simulink model "transystem2"  (Simulink 10.0)
settings: Solver=ode15s  StartTime=0.0  StopTime=1  RelTol=1e-3  AbsTol=1e-6
libraries: powerlib x86, powerlib_extras x4
settings Model: Creator=Dr. Lotfifard  LastModifiedBy=bae_rashid  ExtModeTrigMode=oneshot  ExtModeArmWhenConnect=off
settings SolverCC: AutoScaleAbsTol=off
settings DataIOCC: SignalLoggingSaveFormat=ModelDataLogs
settings OptimizationCC: BlockReduction=off  BooleanDataType=off  ExpressionDepthLimit=2147483647
settings DebuggingCC: SaveWithParameterizedLinksMsg=none  SignalResolutionControl=TryResolveAllWithWarning  MultiTaskDSMMsg=warning  MultiTaskCondExecSysMsg=none  FcnCallInpInsideContextMsg=warning  StateNameClashWarn=warning
settings HardwareCC: TargetUnknown=on
settings GRTTargetCC: GeneratePreprocessorConditionals=Disable all
settings ConfigComp: CovExternalEMLEnable=off
settings SimscapeCC: SimscapeNormalizeSystem=off

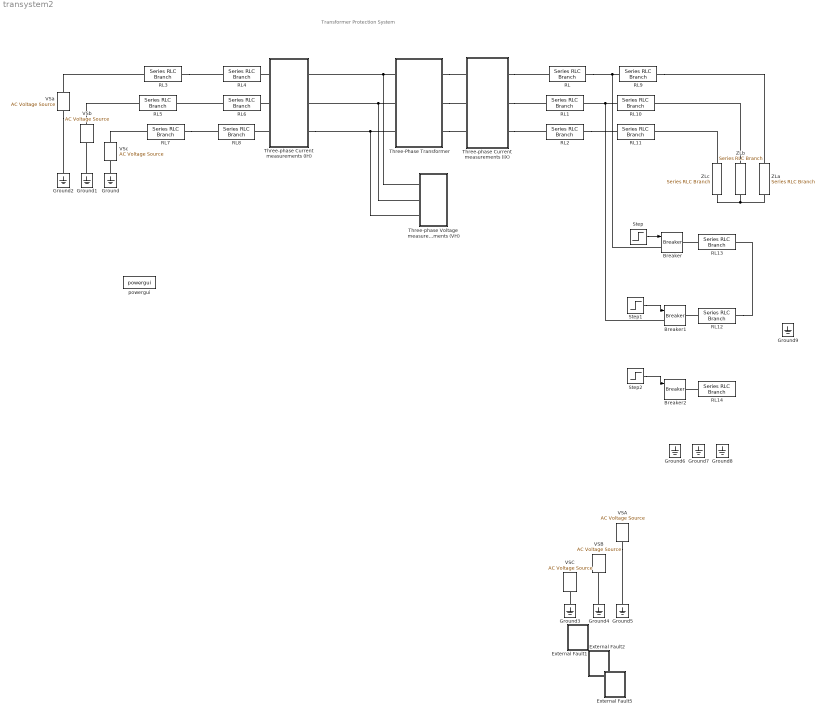
== system transystem2 ==
  note: Transformer Protection System
  Breaker : powerlib/Elements/Breaker  Tag=PoWeRsYsTeMbLoCk  InitialState=0  SwitchingTimes="[ 1/60  5/60 ]"  External=on  BreakerResistance=0.01  SnubberResistance=1e6  SnubberCapacitance=inf  Measurements=None  MoreParameters=off  NoBreakLoop=off
      settings: SourceProductName=Simscape Electrical
  Breaker1 : powerlib/Elements/Breaker  Tag=PoWeRsYsTeMbLoCk  InitialState=0  SwitchingTimes="[ 1/60  5/60 ]"  External=on  BreakerResistance=0.01  SnubberResistance=1e6  SnubberCapacitance=inf  Measurements=None  MoreParameters=off  NoBreakLoop=off
      settings: SourceProductName=Simscape Electrical
  Breaker2 : powerlib/Elements/Breaker  Tag=PoWeRsYsTeMbLoCk  InitialState=0  SwitchingTimes="[ 1/60  5/60 ]"  External=on  BreakerResistance=0.01  SnubberResistance=1e6  SnubberCapacitance=inf  Measurements=None  MoreParameters=off  NoBreakLoop=off
      settings: SourceProductName=Simscape Electrical
  External Fault1 : Subsystem  mask(Fault){RF=1, tf=0.5}
      mask prompts: RF "Resistance [ohm]"; tf "Time [sec]"
      mask Display: plot(0,0,100,100,[44,47,56,38,50],[23,8,64,44,97],[56,47],[25,8])
  External Fault2 : Subsystem  mask(Fault){RF=1, tf=0.5}
      mask prompts: RF "Resistance [ohm]"; tf "Time [sec]"
      mask Display: plot(0,0,100,100,[44,47,56,38,50],[23,8,64,44,97],[56,47],[25,8])
  External Fault5 : Subsystem  mask(Fault){RF=1, tf=0.5}
      mask prompts: RF "Resistance [ohm]"; tf "Time [sec]"
      mask Display: plot(0,0,100,100,[44,47,56,38,50],[23,8,64,44,97],[56,47],[25,8])
  Ground{,1..9} (10 alike) : powerlib/Elements/Ground  LConnTagsString=a
      settings: SourceProductName=Simscape Electrical
  RL{,1..2,9..11} (6 alike) : powerlib/Elements/Series RLC Branch  LConnTagsString=__new0  RConnTagsString=__new0  BranchType=RL  Resistance=10  Inductance=0.033  SetiL0=off  InitialCurrent=0  Capacitance=1e-6  Setx0=off  InitialVoltage=0  Measurements=None
      settings: SourceProductName=Simscape Electrical
  RL12 : powerlib/Elements/Series RLC Branch  LConnTagsString=__new0  RConnTagsString=__new0  BranchType=RL  Resistance=1  Inductance=0.000001/(2*pi*60)/(2*pi*60)  SetiL0=off  InitialCurrent=0  Capacitance=1e-6  Setx0=off  InitialVoltage=0  Measurements=None
      settings: SourceProductName=Simscape Electrical
  RL13 : powerlib/Elements/Series RLC Branch  LConnTagsString=__new0  RConnTagsString=__new0  BranchType=RL  Resistance=1  Inductance=0.000001/(2*pi*60)  SetiL0=off  InitialCurrent=0  Capacitance=1e-6  Setx0=off  InitialVoltage=0  Measurements=None
      settings: SourceProductName=Simscape Electrical
  RL14 : powerlib/Elements/Series RLC Branch  LConnTagsString=__new0  RConnTagsString=__new0  BranchType=RL  Resistance=1  Inductance=0.000001/(2*pi*60)/(2*pi*60)  SetiL0=off  InitialCurrent=0  Capacitance=1e-6  Setx0=off  InitialVoltage=0  Measurements=None
      settings: SourceProductName=Simscape Electrical
  RL{3..8} (6 alike) : powerlib/Elements/Series RLC Branch  LConnTagsString=__new0  RConnTagsString=__new0  BranchType=RL  Resistance=6  Inductance=0.09  SetiL0=off  InitialCurrent=0  Capacitance=1e-6  Setx0=off  InitialVoltage=0  Measurements=None
      settings: SourceProductName=Simscape Electrical
  Step : Step  Time=0.5
  Step1 : Step  Time=0.5
  Step2 : Step  Time=0.5
  Three-Phase Transformer : Subsystem
  Three-phase Current  measurements (IH) : Subsystem
  Three-phase Current  measurements (IX) : Subsystem
  Three-phase Voltage  measurements (VH) : Subsystem
  VSA : powerlib/Electrical Sources/AC Voltage Source  Amplitude=3.8e3/sqrt(3)*sqrt(2)  Phase=0  Frequency=60  SampleTime=0  Measurements=None  BusType=swing  Pref=10e3  Qref=0  Qmin=-inf  Qmax=+inf
      settings: SourceProductName=Simscape Electrical
  VSB : powerlib/Electrical Sources/AC Voltage Source  Amplitude=3.8e3/sqrt(3)*sqrt(2)  Phase=-120  Frequency=60  SampleTime=0  Measurements=None  BusType=swing  Pref=10e3  Qref=0  Qmin=-inf  Qmax=+inf
      settings: SourceProductName=Simscape Electrical
  VSC : powerlib/Electrical Sources/AC Voltage Source  Amplitude=3.8e3/sqrt(3)*sqrt(2)  Phase=120  Frequency=60  SampleTime=0  Measurements=None  BusType=swing  Pref=10e3  Qref=0  Qmin=-inf  Qmax=+inf
      settings: SourceProductName=Simscape Electrical
  VSa : powerlib/Electrical Sources/AC Voltage Source  Amplitude=315e3/sqrt(3)*sqrt(2)  Phase=0  Frequency=60  SampleTime=0  Measurements=None  BusType=swing  Pref=10e3  Qref=0  Qmin=-inf  Qmax=+inf
      settings: SourceProductName=Simscape Electrical
  VSb : powerlib/Electrical Sources/AC Voltage Source  Amplitude=315e3/sqrt(3)*sqrt(2)  Phase=-120  Frequency=60  SampleTime=0  Measurements=None  BusType=swing  Pref=10e3  Qref=0  Qmin=-inf  Qmax=+inf
      settings: SourceProductName=Simscape Electrical
  VSc : powerlib/Electrical Sources/AC Voltage Source  Amplitude=315e3/sqrt(3)*sqrt(2)  Phase=120  Frequency=60  SampleTime=0  Measurements=None  BusType=swing  Pref=10e3  Qref=0  Qmin=-inf  Qmax=+inf
      settings: SourceProductName=Simscape Electrical
  ZLa : powerlib/Elements/Series RLC Branch  LConnTagsString=__new0  RConnTagsString=__new0  BranchType=RL  Resistance=300  Inductance=450/(2*pi*60)  SetiL0=off  InitialCurrent=0  Capacitance=1.0  Setx0=off  InitialVoltage=0  Measurements=None
      settings: SourceProductName=Simscape Electrical
  ZLb : powerlib/Elements/Series RLC Branch  LConnTagsString=__new0  RConnTagsString=__new0  BranchType=RL  Resistance=300  Inductance=450/(2*pi*60)  SetiL0=off  InitialCurrent=0  Capacitance=1.0  Setx0=off  InitialVoltage=0  Measurements=None
      settings: SourceProductName=Simscape Electrical
  ZLc : powerlib/Elements/Series RLC Branch  LConnTagsString=__new0  RConnTagsString=__new0  BranchType=RL  Resistance=300  Inductance=450/(2*pi*60)  SetiL0=off  InitialCurrent=0  Capacitance=1.0  Setx0=off  InitialVoltage=0  Measurements=None
      settings: SourceProductName=Simscape Electrical
  powergui : powerlib/powergui  SimulationMode=Continuous  SampleTime=0  frequency=60  Iterations=50  frequencyindice=60  Pbase=100e6  ErrMax=1e-4  UnitsV=kV  UnitsW=MW  buscounter=0  FunctionMessages=off  echomessages=off  EnableUseOfTLC=off  CurrentSourceSwitches=on  DisableSnubberDevices=off  DisableRonSwitches=off  DisableVfSwitches=off  DisplayEquations=off  AutomaticDiscreteSolvers=off  SolverType=Tustin/Backward Euler (TBE)  Interpol=off  ExternalGateDelay=off  methode=off  Ts=0  x0status=blocks  SPID=off  SwTol=0  HookPort=off  NonlinearTolerance=0  nMaxIteration=15  ContinueOnMaxIteration=off  RestoreLinks=warning  ResistiveCurrentMeasurement=off  Frange=[0:2:500]  Ylog=off  Xlog=on  ShowGrid=off  save=off  variable=ZData  structure=0  ZoomFFT=on  StartTime=0.0  cycles=1  DisplayStyle=1  fundamental=60  FreqAxis=off  MaxFrequency=1000  frequencyindicesteady=1  RmsSteady=1  display=off
      settings: SourceProductName=Simscape Electrical
  wires:
  Step/1 -> Breaker/1
  Step1/1 -> Breaker1/1
  Step2/1 -> Breaker2/1
  connections:
  Ground/LConn1 -- VSc/LConn1
  Ground1/LConn1 -- VSb/LConn1
  VSa/LConn1 -- Ground2/LConn1
  RL5/LConn1 -- VSb/RConn1
  Three-phase Current  measurements (IH)/LConn2 -- RL6/RConn1
  Three-phase Current  measurements (IH)/LConn3 -- RL8/RConn1
  Three-phase Current  measurements (IH)/LConn1 -- RL4/RConn1
  VSa/RConn1 -- RL3/LConn1
  RL6/LConn1 -- RL5/RConn1
  RL3/RConn1 -- RL4/LConn1
  RL7/RConn1 -- RL8/LConn1
  RL7/LConn1 -- VSc/RConn1
  RL10/LConn1 -- Breaker1/LConn1 -- RL1/RConn1
  RL/RConn1 -- Breaker/LConn1 -- RL9/LConn1
  RL2/RConn1 -- RL11/LConn1
  Ground3/LConn1 -- VSC/LConn1
  Ground4/LConn1 -- VSB/LConn1
  VSA/LConn1 -- Ground5/LConn1
  Three-Phase Transformer/LConn2 -- Three-phase Current  measurements (IH)/RConn2 -- Three-phase Voltage  measurements (VH)/LConn2
  Three-Phase Transformer/LConn1 -- Three-phase Current  measurements (IH)/RConn1 -- Three-phase Voltage  measurements (VH)/LConn1
  Three-Phase Transformer/RConn1 -- Three-phase Current  measurements (IX)/LConn1
  Three-phase Current  measurements (IH)/RConn3 -- Three-Phase Transformer/LConn3 -- Three-phase Voltage  measurements (VH)/LConn3
  Three-Phase Transformer/RConn3 -- Three-phase Current  measurements (IX)/LConn3
  Three-Phase Transformer/RConn2 -- Three-phase Current  measurements (IX)/LConn2
  ZLc/RConn1 -- ZLa/RConn1 -- ZLb/RConn1
  Three-phase Current  measurements (IX)/RConn3 -- RL2/LConn1
  Three-phase Current  measurements (IX)/RConn2 -- RL1/LConn1
  Three-phase Current  measurements (IX)/RConn1 -- RL/LConn1
  ZLb/LConn1 -- RL10/RConn1
  ZLc/LConn1 -- RL11/RConn1
  RL9/RConn1 -- ZLa/LConn1
  RL13/LConn1 -- Breaker/RConn1
  RL12/LConn1 -- Breaker1/RConn1
  RL14/LConn1 -- Breaker2/RConn1
  RL12/RConn1 -- RL13/RConn1

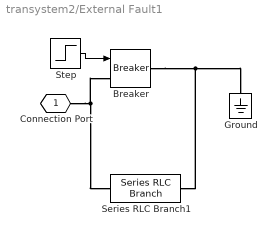
== system transystem2/External Fault1 ==
  Breaker : powerlib/Elements/Breaker  Tag=PoWeRsYsTeMbLoCk  InitialState=0  SwitchingTimes="[ 1/60  5/60 ]"  External=on  BreakerResistance=0.01  SnubberResistance=1e6  SnubberCapacitance=inf  Measurements=None  MoreParameters=off  NoBreakLoop=off
      settings: SourceProductName=Simscape Electrical
  Ground : powerlib/Elements/Ground  LConnTagsString=a
      settings: SourceProductName=Simscape Electrical
  Series RLC Branch1 : powerlib/Elements/Series RLC Branch  LConnTagsString=__new0  RConnTagsString=__new0  BranchType=RLC  Resistance=1  Inductance=1e-3  SetiL0=off  InitialCurrent=0  Capacitance=1e-6  Setx0=off  InitialVoltage=0  Measurements=None
      settings: SourceProductName=Simscape Electrical
  Step : Step  Time=tf
  Connection Port : PMIOPort  Tag=PMCPort  Side=Left
  wires:
  Step/1 -> Breaker/1
  connections:
  Breaker/RConn1 -- Ground/LConn1 -- Series RLC Branch1/RConn1
  Connection Port/RConn1 -- Breaker/LConn1 -- Series RLC Branch1/LConn1

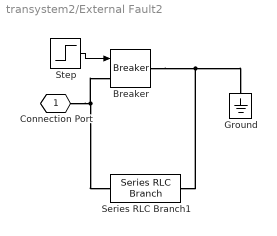
== system transystem2/External Fault2 ==
  Breaker : powerlib/Elements/Breaker  Tag=PoWeRsYsTeMbLoCk  InitialState=0  SwitchingTimes="[ 1/60  5/60 ]"  External=on  BreakerResistance=0.01  SnubberResistance=1e6  SnubberCapacitance=inf  Measurements=None  MoreParameters=off  NoBreakLoop=off
      settings: SourceProductName=Simscape Electrical
  Ground : powerlib/Elements/Ground  LConnTagsString=a
      settings: SourceProductName=Simscape Electrical
  Series RLC Branch1 : powerlib/Elements/Series RLC Branch  LConnTagsString=__new0  RConnTagsString=__new0  BranchType=RLC  Resistance=1  Inductance=1e-3  SetiL0=off  InitialCurrent=0  Capacitance=1e-6  Setx0=off  InitialVoltage=0  Measurements=None
      settings: SourceProductName=Simscape Electrical
  Step : Step  Time=tf
  Connection Port : PMIOPort  Tag=PMCPort  Side=Left
  wires:
  Step/1 -> Breaker/1
  connections:
  Breaker/RConn1 -- Ground/LConn1 -- Series RLC Branch1/RConn1
  Connection Port/RConn1 -- Breaker/LConn1 -- Series RLC Branch1/LConn1

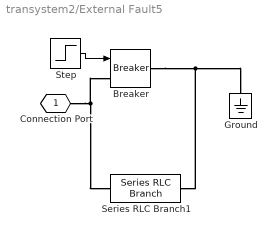
== system transystem2/External Fault5 ==
  Breaker : powerlib/Elements/Breaker  Tag=PoWeRsYsTeMbLoCk  InitialState=0  SwitchingTimes="[ 1/60  5/60 ]"  External=on  BreakerResistance=0.01  SnubberResistance=1e6  SnubberCapacitance=inf  Measurements=None  MoreParameters=off  NoBreakLoop=off
      settings: SourceProductName=Simscape Electrical
  Ground : powerlib/Elements/Ground  LConnTagsString=a
      settings: SourceProductName=Simscape Electrical
  Series RLC Branch1 : powerlib/Elements/Series RLC Branch  LConnTagsString=__new0  RConnTagsString=__new0  BranchType=RLC  Resistance=1  Inductance=1e-3  SetiL0=off  InitialCurrent=0  Capacitance=1e-6  Setx0=off  InitialVoltage=0  Measurements=None
      settings: SourceProductName=Simscape Electrical
  Step : Step  Time=tf
  Connection Port : PMIOPort  Tag=PMCPort  Side=Left
  wires:
  Step/1 -> Breaker/1
  connections:
  Breaker/RConn1 -- Ground/LConn1 -- Series RLC Branch1/RConn1
  Connection Port/RConn1 -- Breaker/LConn1 -- Series RLC Branch1/LConn1

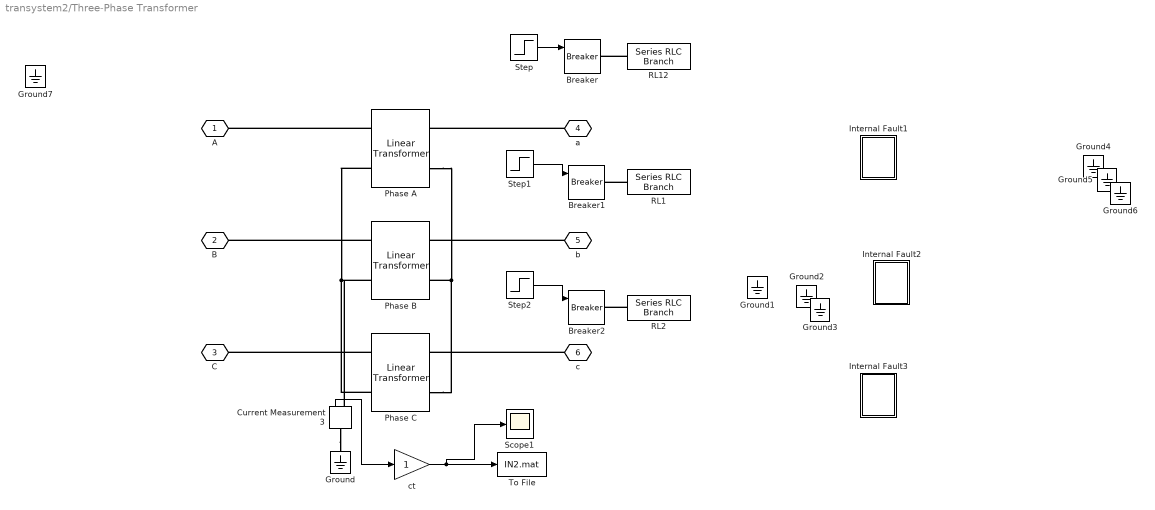
== system transystem2/Three-Phase Transformer ==
  Breaker : powerlib/Elements/Breaker  Tag=PoWeRsYsTeMbLoCk  InitialState=0  SwitchingTimes="[ 1/60  5/60 ]"  External=on  BreakerResistance=0.01  SnubberResistance=1e6  SnubberCapacitance=inf  Measurements=None  MoreParameters=off  NoBreakLoop=off
      settings: SourceProductName=Simscape Electrical
  Breaker1 : powerlib/Elements/Breaker  Tag=PoWeRsYsTeMbLoCk  InitialState=0  SwitchingTimes="[ 1/60  5/60 ]"  External=on  BreakerResistance=0.01  SnubberResistance=1e6  SnubberCapacitance=inf  Measurements=None  MoreParameters=off  NoBreakLoop=off
      settings: SourceProductName=Simscape Electrical
  Breaker2 : powerlib/Elements/Breaker  Tag=PoWeRsYsTeMbLoCk  InitialState=0  SwitchingTimes="[ 1/60  5/60 ]"  External=on  BreakerResistance=0.01  SnubberResistance=1e6  SnubberCapacitance=inf  Measurements=None  MoreParameters=off  NoBreakLoop=off
      settings: SourceProductName=Simscape Electrical
  Current Measurement3 : powerlib/Measurements/Current Measurement  PhasorSimulation=off  OutputType=Complex  PSBequivalent=0
      settings: SourceProductName=Simscape Electrical
  Ground{,1..7} (8 alike) : powerlib/Elements/Ground  LConnTagsString=a
      settings: SourceProductName=Simscape Electrical
  Internal Fault1 : Subsystem  mask(Fault){RF=1, tf=0.5}
      mask prompts: RF "Resistance [ohm]"; tf "Time [sec]"
      mask Display: plot(0,0,100,100,[44,47,56,38,50],[23,8,64,44,97],[56,47],[25,8])
  Internal Fault2 : Subsystem  mask(Fault){RF=1, tf=0.5}
      mask prompts: RF "Resistance [ohm]"; tf "Time [sec]"
      mask Display: plot(0,0,100,100,[44,47,56,38,50],[23,8,64,44,97],[56,47],[25,8])
  Internal Fault3 : Subsystem  mask(Fault){RF=1, tf=0.5}
      mask prompts: RF "Resistance [ohm]"; tf "Time [sec]"
      mask Display: plot(0,0,100,100,[44,47,56,38,50],[23,8,64,44,97],[56,47],[25,8])
  Phase A : powerlib/Elements/Linear Transformer  UNITS=pu  NominalPower=[ 300e6 60 ]  winding1="[ 315e3  0.0025  0.1 ]"  winding2="[ 13.8e3  0.0025  0.1 ]"  ThreeWindings=off  winding3=[ 315e3 0.002 0.08 ]  RmLm=[ 1e6 inf ]  Measurements=None  DataType=off
      settings: SourceProductName=Simscape Electrical
  Phase B : powerlib/Elements/Linear Transformer  UNITS=pu  NominalPower=[ 300e6 60 ]  winding1="[ 315e3  0.0025  0.1 ]"  winding2="[ 13.8e3  0.0025  0.1 ]"  ThreeWindings=off  winding3=[ 315e3 0.002 0.08 ]  RmLm=[ 1e6 inf ]  Measurements=None  DataType=off
      settings: SourceProductName=Simscape Electrical
  Phase C : powerlib/Elements/Linear Transformer  UNITS=pu  NominalPower=[ 300e6 60 ]  winding1="[ 315e3  0.0025  0.1 ]"  winding2="[ 13.8e3  0.0025  0.1 ]"  ThreeWindings=off  winding3=[ 315e3 0.002 0.08 ]  RmLm=[1e6 inf ]  Measurements=None  DataType=off
      settings: SourceProductName=Simscape Electrical
  RL1 : powerlib/Elements/Series RLC Branch  LConnTagsString=__new0  RConnTagsString=__new0  BranchType=RL  Resistance=1.5  Inductance=2/(2*pi*60)  SetiL0=off  InitialCurrent=0  Capacitance=1e-6  Setx0=off  InitialVoltage=0  Measurements=None
      settings: SourceProductName=Simscape Electrical
  RL12 : powerlib/Elements/Series RLC Branch  LConnTagsString=__new0  RConnTagsString=__new0  BranchType=RL  Resistance=1.5  Inductance=2/(2*pi*60)  SetiL0=off  InitialCurrent=0  Capacitance=1e-6  Setx0=off  InitialVoltage=0  Measurements=None
      settings: SourceProductName=Simscape Electrical
  RL2 : powerlib/Elements/Series RLC Branch  LConnTagsString=__new0  RConnTagsString=__new0  BranchType=RL  Resistance=1.5  Inductance=2/(2*pi*60)  SetiL0=off  InitialCurrent=0  Capacitance=1e-6  Setx0=off  InitialVoltage=0  Measurements=None
      settings: SourceProductName=Simscape Electrical
  Scope1 : Scope
  Step : Step  Time=0.5
  Step1 : Step  Time=0.5
  Step2 : Step  Time=0.5
  To File : ToFile  Filename=IN2.mat  MatrixName=iha
  ct : Gain  SaturateOnIntegerOverflow=on  OutDataTypeStr=Inherit: Same as input  ParamDataTypeStr=Inherit: Same as input
  A : PMIOPort  Tag=PMCPort  Side=Left
  B : PMIOPort  Tag=PMCPort  Port=2  Side=Left
  C : PMIOPort  Tag=PMCPort  Port=3  Side=Left
  a : PMIOPort  Tag=PMCPort  Port=4  Side=Right
  b : PMIOPort  Tag=PMCPort  Port=5  Side=Right
  c : PMIOPort  Tag=PMCPort  Port=6  Side=Right
  wires:
  ct/1 -> Scope1/1, To File/1
  Current Measurement3/1 -> ct/1
  Step/1 -> Breaker/1
  Step1/1 -> Breaker1/1
  Step2/1 -> Breaker2/1
  connections:
  b/RConn1 -- Phase B/RConn1
  Phase B/LConn1 -- B/RConn1
  c/RConn1 -- Phase C/RConn1
  Phase B/LConn2 -- Current Measurement3/RConn1 -- Phase C/LConn2 -- Phase A/LConn2
  a/RConn1 -- Phase A/RConn1
  Phase C/LConn1 -- C/RConn1
  Phase A/LConn1 -- A/RConn1
  Current Measurement3/LConn1 -- Ground/LConn1
  Phase A/RConn2 -- Phase C/RConn2 -- Phase B/RConn2
  RL12/LConn1 -- Breaker/RConn1
  RL1/LConn1 -- Breaker1/RConn1
  RL2/LConn1 -- Breaker2/RConn1

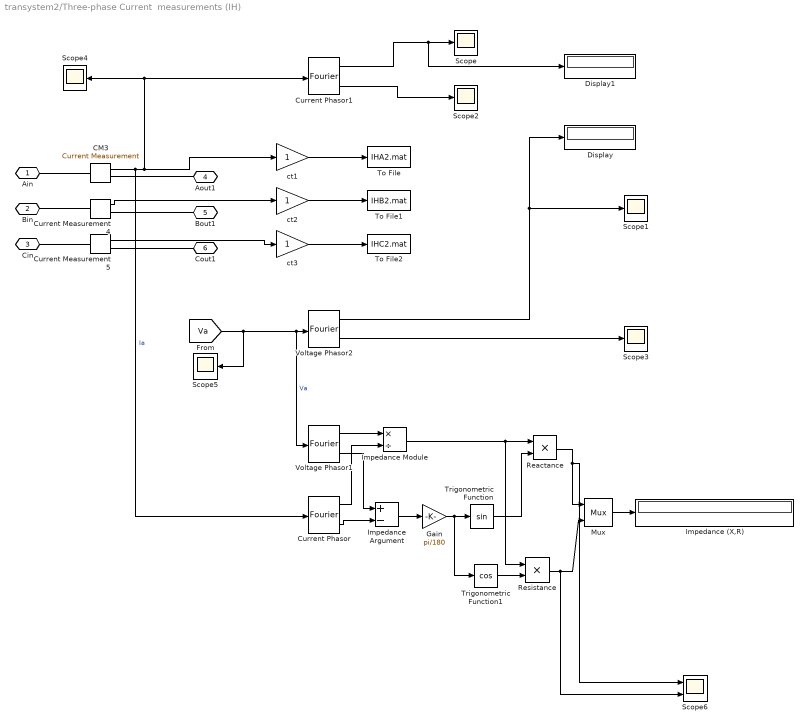
== system transystem2/Three-phase Current  measurements (IH) ==
  CM3 : powerlib/Measurements/Current Measurement  PhasorSimulation=off  OutputType=Complex  PSBequivalent=0
      settings: SourceProductName=Simscape Electrical
  Current Phasor : powerlib_extras/Measurements/Fourier  f1=60  n=1
      settings: SourceProductName=Simscape Electrical  SourceProductBaseCode=PS
  Current Phasor1 : powerlib_extras/Measurements/Fourier  f1=60  n=1
      settings: SourceProductName=Simscape Electrical  SourceProductBaseCode=PS
  Current Measurement4 : powerlib/Measurements/Current Measurement  PhasorSimulation=off  OutputType=Complex  PSBequivalent=0
      settings: SourceProductName=Simscape Electrical
  Current Measurement5 : powerlib/Measurements/Current Measurement  PhasorSimulation=off  OutputType=Complex  PSBequivalent=0
      settings: SourceProductName=Simscape Electrical
  Display : Display
      settings: Format=bank  Decimation=2
  Display1 : Display
      settings: Decimation=2
  Gain : Gain  Gain=pi/180  SaturateOnIntegerOverflow=on  OutDataTypeStr=Inherit: Same as input  ParamDataTypeStr=Inherit: Same as input
  Impedance Argument : Sum  Inputs=+-  SaturateOnIntegerOverflow=on  InputSameDT=on  OutDataTypeStr=Inherit: Same as first input
  Impedance Module : Product  Inputs=*/  SaturateOnIntegerOverflow=on  RndMeth=Zero  InputSameDT=on  OutDataTypeStr=Inherit: Same as first input
  Impedance (X,R) : Display
      settings: Format=bank
  Mux : Mux  Inputs=2
  Reactance : Product  Inputs=**  SaturateOnIntegerOverflow=on  RndMeth=Zero  InputSameDT=on  OutDataTypeStr=Inherit: Same as first input
  Resistance : Product  Inputs=**  SaturateOnIntegerOverflow=on  RndMeth=Zero  InputSameDT=on  OutDataTypeStr=Inherit: Same as first input
  Scope{,1..5} (6 alike) : Scope
  Scope6 : Scope  NumInputPorts=2
  To File : ToFile  Filename=IHA2.mat  MatrixName=iha
  To File1 : ToFile  Filename=IHB2.mat  MatrixName=ihb
  To File2 : ToFile  Filename=IHC2.mat  MatrixName=ihc
  Trigonometric Function : Trigonometry
  Trigonometric Function1 : Trigonometry  Operator=cos
  Voltage Phasor1 : powerlib_extras/Measurements/Fourier  f1=60  n=1
      settings: SourceProductName=Simscape Electrical  SourceProductBaseCode=PS
  Voltage Phasor2 : powerlib_extras/Measurements/Fourier  f1=60  n=1
      settings: SourceProductName=Simscape Electrical  SourceProductBaseCode=PS
  ct1 : Gain  SaturateOnIntegerOverflow=on  OutDataTypeStr=Inherit: Same as input  ParamDataTypeStr=Inherit: Same as input
  ct2 : Gain  SaturateOnIntegerOverflow=on  OutDataTypeStr=Inherit: Same as input  ParamDataTypeStr=Inherit: Same as input
  ct3 : Gain  SaturateOnIntegerOverflow=on  OutDataTypeStr=Inherit: Same as input  ParamDataTypeStr=Inherit: Same as input
  Ain : PMIOPort  Side=Left
  Bin : PMIOPort  Port=2  Side=Left
  Cin : PMIOPort  Port=3  Side=Left
  Aout1 : PMIOPort  Port=4  Side=Right
  Bout1 : PMIOPort  Port=5  Side=Right
  Cout1 : PMIOPort  Port=6  Side=Right
  wires:
  ct2/1 -> To File1/1
  ct3/1 -> To File2/1
  Current Measurement4/1 -> ct2/1
  Current Measurement5/1 -> ct3/1
  ct1/1 -> To File/1
  CM3/1 -> Current Phasor/1, Scope4/1, Current Phasor1/1, ct1/1  "Ia"
  Current Phasor1/1 -> Display1/1, Scope/1
  Current Phasor1/2 -> Scope2/1
  Resistance/1 -> Scope6/2, Mux/2
  Current Phasor/1 -> Impedance Module/2
  Mux/1 -> Impedance (X,R)/1
  Current Phasor/2 -> Impedance Argument/2
  Trigonometric Function1/1 -> Resistance/2
  Impedance Argument/1 -> Gain/1
  Voltage Phasor1/2 -> Impedance Argument/1
  Impedance Module/1 -> Reactance/1, Resistance/1
  Trigonometric Function/1 -> Reactance/2
  Gain/1 -> Trigonometric Function/1, Trigonometric Function1/1
  Reactance/1 -> Scope6/1, Mux/1
  Voltage Phasor1/1 -> Impedance Module/1
  [Va] -> Scope5/1, Voltage Phasor1/1, Voltage Phasor2/1  "Va"
  Voltage Phasor2/1 -> Display/1, Scope1/1
  Voltage Phasor2/2 -> Scope3/1
  connections:
  Current Measurement4/RConn1 -- Bout1/RConn1
  CM3/LConn1 -- Ain/RConn1
  Current Measurement5/LConn1 -- Cin/RConn1
  CM3/RConn1 -- Aout1/RConn1
  Current Measurement4/LConn1 -- Bin/RConn1
  Current Measurement5/RConn1 -- Cout1/RConn1

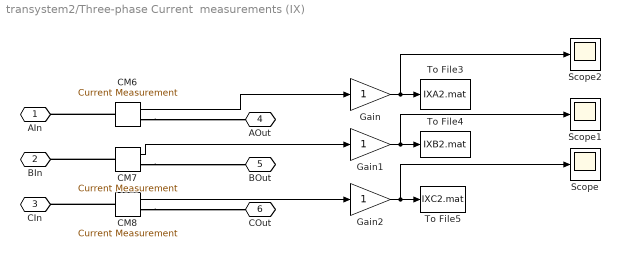
== system transystem2/Three-phase Current  measurements (IX) ==
  CM6 : powerlib/Measurements/Current Measurement  PhasorSimulation=off  OutputType=Complex  PSBequivalent=0
      settings: SourceProductName=Simscape Electrical
  CM7 : powerlib/Measurements/Current Measurement  PhasorSimulation=off  OutputType=Complex  PSBequivalent=0
      settings: SourceProductName=Simscape Electrical
  CM8 : powerlib/Measurements/Current Measurement  PhasorSimulation=off  OutputType=Complex  PSBequivalent=0
      settings: SourceProductName=Simscape Electrical
  Gain : Gain  SaturateOnIntegerOverflow=on  OutDataTypeStr=Inherit: Same as input  ParamDataTypeStr=Inherit: Same as input
  Gain1 : Gain  SaturateOnIntegerOverflow=on  OutDataTypeStr=Inherit: Same as input  ParamDataTypeStr=Inherit: Same as input
  Gain2 : Gain  SaturateOnIntegerOverflow=on  OutDataTypeStr=Inherit: Same as input  ParamDataTypeStr=Inherit: Same as input
  Scope : Scope
  Scope1 : Scope
  Scope2 : Scope
  To File3 : ToFile  Filename=IXA2.mat  MatrixName=ixa
  To File4 : ToFile  Filename=IXB2.mat  MatrixName=ixb
  To File5 : ToFile  Filename=IXC2.mat  MatrixName=ixc
  AIn : PMIOPort  Side=Left
  BIn : PMIOPort  Port=2  Side=Left
  CIn : PMIOPort  Port=3  Side=Left
  AOut : PMIOPort  Port=4  Side=Right
  BOut : PMIOPort  Port=5  Side=Right
  COut : PMIOPort  Port=6  Side=Right
  wires:
  Gain2/1 -> To File5/1, Scope/1
  Gain1/1 -> To File4/1, Scope1/1
  Gain/1 -> To File3/1, Scope2/1
  CM7/1 -> Gain1/1
  CM6/1 -> Gain/1
  CM8/1 -> Gain2/1
  connections:
  CM7/RConn1 -- BOut/RConn1
  CM6/LConn1 -- AIn/RConn1
  CM6/RConn1 -- AOut/RConn1
  CM8/RConn1 -- COut/RConn1
  CM7/LConn1 -- BIn/RConn1
  CM8/LConn1 -- CIn/RConn1

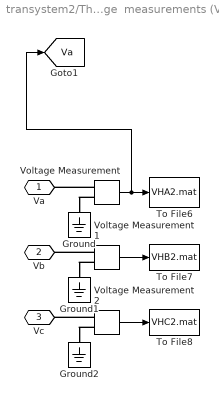
== system transystem2/Three-phase Voltage  measurements (VH) ==
  Ground : powerlib/Elements/Ground  LConnTagsString=a
      settings: SourceProductName=Simscape Electrical
  Ground1 : powerlib/Elements/Ground  LConnTagsString=a
      settings: SourceProductName=Simscape Electrical
  Ground2 : powerlib/Elements/Ground  LConnTagsString=a
      settings: SourceProductName=Simscape Electrical
  To File6 : ToFile  Filename=VHA2.mat  MatrixName=vha
  To File7 : ToFile  Filename=VHB2.mat  MatrixName=vhb
  To File8 : ToFile  Filename=VHC2.mat  MatrixName=vhc
  Voltage Measurement : powerlib/Measurements/Voltage Measurement  PhasorSimulation=off  OutputType=Complex  PSBequivalent=0
      settings: SourceProductName=Simscape Electrical
  Voltage Measurement1 : powerlib/Measurements/Voltage Measurement  PhasorSimulation=off  OutputType=Complex  PSBequivalent=0
      settings: SourceProductName=Simscape Electrical
  Voltage Measurement2 : powerlib/Measurements/Voltage Measurement  PhasorSimulation=off  OutputType=Complex  PSBequivalent=0
      settings: SourceProductName=Simscape Electrical
  Va : PMIOPort  Side=Left
  Vb : PMIOPort  Port=2  Side=Left
  Vc : PMIOPort  Port=3  Side=Left
  tag scope: Va=global
  wires:
  Voltage Measurement/1 -> [Va], To File6/1
  Voltage Measurement1/1 -> To File7/1
  Voltage Measurement2/1 -> To File8/1
  connections:
  Voltage Measurement/LConn2 -- Ground/LConn1
  Voltage Measurement1/LConn2 -- Ground1/LConn1
  Voltage Measurement2/LConn2 -- Ground2/LConn1
  Voltage Measurement2/LConn1 -- Vc/RConn1
  Voltage Measurement1/LConn1 -- Vb/RConn1
  Voltage Measurement/LConn1 -- Va/RConn1

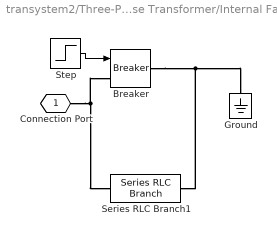
== system transystem2/Three-Phase Transformer/Internal Fault1 ==
  Breaker : powerlib/Elements/Breaker  Tag=PoWeRsYsTeMbLoCk  InitialState=0  SwitchingTimes="[ 1/60  5/60 ]"  External=on  BreakerResistance=0.01  SnubberResistance=1e6  SnubberCapacitance=inf  Measurements=None  MoreParameters=off  NoBreakLoop=off
      settings: SourceProductName=Simscape Electrical
  Ground : powerlib/Elements/Ground  LConnTagsString=a
      settings: SourceProductName=Simscape Electrical
  Series RLC Branch1 : powerlib/Elements/Series RLC Branch  LConnTagsString=__new0  RConnTagsString=__new0  BranchType=RLC  Resistance=1  Inductance=1e-3  SetiL0=off  InitialCurrent=0  Capacitance=1e-6  Setx0=off  InitialVoltage=0  Measurements=None
      settings: SourceProductName=Simscape Electrical
  Step : Step  Time=tf
  Connection Port : PMIOPort  Tag=PMCPort  Side=Left
  wires:
  Step/1 -> Breaker/1
  connections:
  Breaker/RConn1 -- Ground/LConn1 -- Series RLC Branch1/RConn1
  Connection Port/RConn1 -- Breaker/LConn1 -- Series RLC Branch1/LConn1

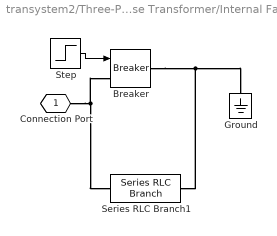
== system transystem2/Three-Phase Transformer/Internal Fault2 ==
  Breaker : powerlib/Elements/Breaker  Tag=PoWeRsYsTeMbLoCk  InitialState=0  SwitchingTimes="[ 1/60  5/60 ]"  External=on  BreakerResistance=0.01  SnubberResistance=1e6  SnubberCapacitance=inf  Measurements=None  MoreParameters=off  NoBreakLoop=off
      settings: SourceProductName=Simscape Electrical
  Ground : powerlib/Elements/Ground  LConnTagsString=a
      settings: SourceProductName=Simscape Electrical
  Series RLC Branch1 : powerlib/Elements/Series RLC Branch  LConnTagsString=__new0  RConnTagsString=__new0  BranchType=RLC  Resistance=1  Inductance=1e-3  SetiL0=off  InitialCurrent=0  Capacitance=1e-6  Setx0=off  InitialVoltage=0  Measurements=None
      settings: SourceProductName=Simscape Electrical
  Step : Step  Time=tf
  Connection Port : PMIOPort  Tag=PMCPort  Side=Left
  wires:
  Step/1 -> Breaker/1
  connections:
  Breaker/RConn1 -- Ground/LConn1 -- Series RLC Branch1/RConn1
  Connection Port/RConn1 -- Breaker/LConn1 -- Series RLC Branch1/LConn1

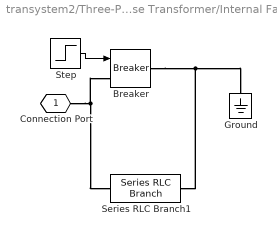
== system transystem2/Three-Phase Transformer/Internal Fault3 ==
  Breaker : powerlib/Elements/Breaker  Tag=PoWeRsYsTeMbLoCk  InitialState=0  SwitchingTimes="[ 1/60  5/60 ]"  External=on  BreakerResistance=0.01  SnubberResistance=1e6  SnubberCapacitance=inf  Measurements=None  MoreParameters=off  NoBreakLoop=off
      settings: SourceProductName=Simscape Electrical
  Ground : powerlib/Elements/Ground  LConnTagsString=a
      settings: SourceProductName=Simscape Electrical
  Series RLC Branch1 : powerlib/Elements/Series RLC Branch  LConnTagsString=__new0  RConnTagsString=__new0  BranchType=RLC  Resistance=1  Inductance=1e-3  SetiL0=off  InitialCurrent=0  Capacitance=1e-6  Setx0=off  InitialVoltage=0  Measurements=None
      settings: SourceProductName=Simscape Electrical
  Step : Step  Time=tf
  Connection Port : PMIOPort  Tag=PMCPort  Side=Left
  wires:
  Step/1 -> Breaker/1
  connections:
  Breaker/RConn1 -- Ground/LConn1 -- Series RLC Branch1/RConn1
  Connection Port/RConn1 -- Breaker/LConn1 -- Series RLC Branch1/LConn1
